simulink model "fuzzy_control"  (R2024a)
settings: Solver=VariableStepAuto  StartTime=0.0  StopTime=10  RelTol=1e-3
libraries: fuzblock x2, simulink x1
settings Model: Creator=ericliu  LastModifiedBy=Eason

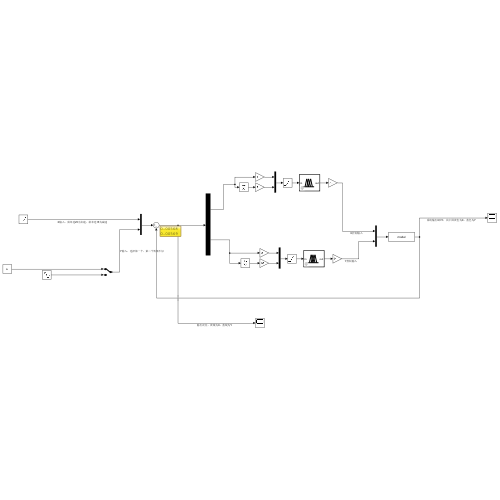
[thumbnail: Simulink's stored preview of the top-level diagram]
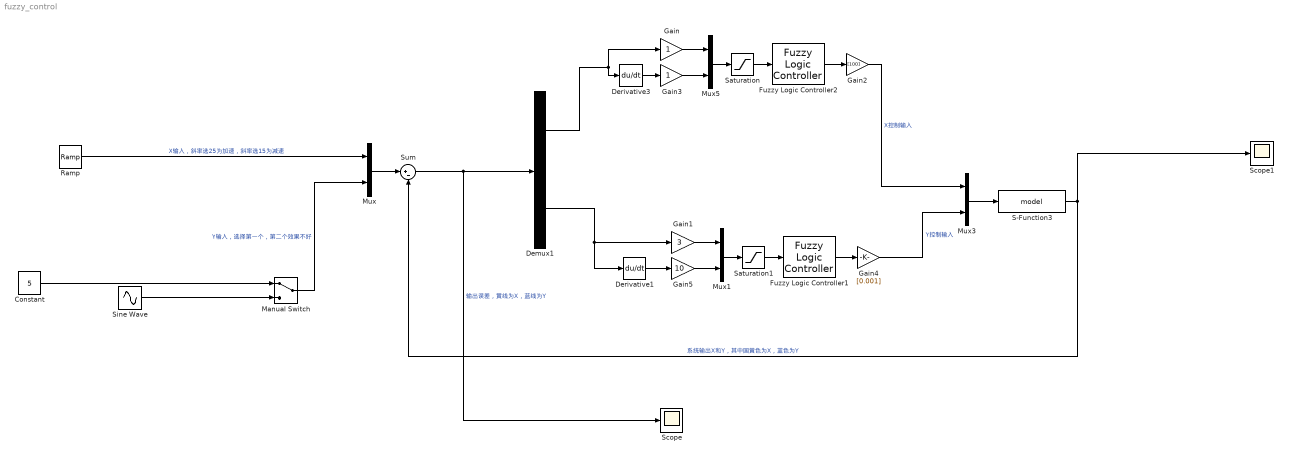
== system fuzzy_control ==
  Constant : Constant  Value=5
  Demux1 : Demux  Outputs=2
  Derivative1 : Derivative
  Derivative3 : Derivative
  Fuzzy Logic Controller1 : fuzblock/Fuzzy Logic  Controller  FIS='fuzzy_direct.fis'  OutputSampleNumber=101  DataType=double  FuzzifiedInputs=off  RuleFiringStrengths=off  RuleOutputs=off  AggregatedOutputs=off  SimulateUsing=Interpreted execution  OutOfRangeInputValueMessage=warning  NoRuleFiredMessage=warning  EmptyOutputFuzzySetMessage=warning
  Fuzzy Logic Controller2 : fuzblock/Fuzzy Logic  Controller  FIS='fuzzy_direct.fis'  OutputSampleNumber=101  DataType=double  FuzzifiedInputs=off  RuleFiringStrengths=off  RuleOutputs=off  AggregatedOutputs=off  SimulateUsing=Interpreted execution  OutOfRangeInputValueMessage=warning  NoRuleFiredMessage=warning  EmptyOutputFuzzySetMessage=warning
  Gain : Gain
  Gain1 : Gain  Gain=3
  Gain2 : Gain  Gain=[100]
  Gain3 : Gain
  Gain4 : Gain  Gain=[0.001]
  Gain5 : Gain  Gain=10
  Manual Switch : ManualSwitch
  Mux{,1,3,5} (4 alike) : Mux  Inputs=2
  Ramp : simulink/Sources/Ramp  slope=25  start=0  InitialOutput=0  VectorParams1D=off
  S-Function3 : S-Function  FunctionName=model  SFunctionDeploymentMode=off  EnableBusSupport=off
  Saturation : Saturate  UpperLimit=10  LowerLimit=-10
  Saturation1 : Saturate  UpperLimit=10  LowerLimit=-10
  Scope : Scope
  Scope1 : Scope
  Sine Wave : Sin  Amplitude=4  Frequency=0.5  SampleTime=0
  Sum : Sum  Inputs=|+-
  wires:
  Sum/1 -> Scope/1, Demux1/1  "输出误差，黄线为X，蓝线为Y"
  Mux/1 -> Sum/1
  Manual Switch/1 -> Mux/2  "Y输入，选择第一个，第二个效果不好"
  Ramp/1 -> Mux/1  "X输入，斜率选25为加速，斜率选15为减速"
  Demux1/1 -> Gain/1, Derivative3/1
  S-Function3/1 -> Sum/2, Scope1/1  "系统输出X和Y，其中国黄色为X，蓝色为Y"
  Derivative3/1 -> Gain3/1
  Mux5/1 -> Saturation/1
  Fuzzy Logic Controller2/1 -> Gain2/1
  Gain2/1 -> Mux3/1  "X控制输入"
  Mux3/1 -> S-Function3/1
  Saturation/1 -> Fuzzy Logic Controller2/1
  Gain/1 -> Mux5/1
  Gain3/1 -> Mux5/2
  Gain1/1 -> Mux1/1
  Fuzzy Logic Controller1/1 -> Gain4/1
  Mux1/1 -> Saturation1/1
  Saturation1/1 -> Fuzzy Logic Controller1/1
  Demux1/2 -> Gain1/1, Derivative1/1
  Gain5/1 -> Mux1/2
  Derivative1/1 -> Gain5/1
  Gain4/1 -> Mux3/2  "Y控制输入"
  Constant/1 -> Manual Switch/1
  Sine Wave/1 -> Manual Switch/2
